simulink model "variableFrequencyConverter"  (R2021b)
settings: Solver=ode23tb  StartTime=simCtrl.startTime  StopTime=simCtrl.endTime  FixedStep=5e-7  RelTol=1e-3  EnableMultiTasking=on
values from neighbouring files (symbols this model uses):
  PhaseA_Grid_Amplitude = sqrt(2)*Vnet / sqrt(3)    [init.m]
  PhaseA_Grid_Bias = 0    [init.m]
  PhaseA_Grid_Frequency = 2*pi*fnet    [init.m]
  PhaseA_Grid_Phase = 0    [init.m]
  PhaseB_Grid_Amplitude = sqrt(2)*Vnet / sqrt(3)    [init.m]
  PhaseB_Grid_Bias = 0    [init.m]
  PhaseB_Grid_Frequency = 2*pi*fnet    [init.m]
  PhaseB_Grid_Phase = -2*pi/3    (= -2.09439510239)    [init.m]
  PhaseC_Grid_Amplitude = sqrt(2)*Vnet / sqrt(3)    [init.m]
  PhaseC_Grid_Bias = 0    [init.m]
  PhaseC_Grid_Frequency = 2*pi*fnet    [init.m]
  PhaseC_Grid_Phase = -4*pi/3    (= -4.18879020479)    [init.m]
  R_Convergence = (motor.un*1000)/(motor.In*sqrt(2))    [init.m]
  TcuP = -1 * TcuP    (= 0)    [init.m]
  TlinP = -1 * TlinP    (= 0)    [init.m]
  TsqP = -1 * TsqP    (= -1)    [init.m]
undefined symbols (not defined in the file or in its folder): ctrl, motor
libraries: spsDiodeLib x6, spsIGBTDiodeLib x6, powerlib_extras x4, spsSeriesRLCBranchLib x4, spsVoltageMeasurementLib x4, spsControlledVoltageSourceLib x3, spsControlledCurrentSourceLib x3, simulink x3, spsThreePhaseVIMeasurementLib x3, spsGroundLib x1, spsTriangleGeneratorLib x1, spspowerguiLib x1
settings Model: ModifiedByFormat=Aravindh Vishnu  Creator=Aravindh Vishnu  LastModifiedBy=Aravindh Vishnu
settings SolverCC: AlgebraicLoopSolver=TrustRegion
settings DataIOCC: FinalStateName=state_p3  InitialState=state_p3  SaveFormat=Array  SignalLoggingSaveFormat=ModelDataLogs  SaveOutput=off  SignalLogging=off  SaveTime=off  ReturnWorkspaceOutputs=off  SignalLoggingName=sigsOut
settings OptimizationCC: BlockReduction=off  DefaultParameterBehavior=Inlined  InlineInvariantSignals=on  BufferReuse=off  ExpressionDepthLimit=2147483647  InitFltsAndDblsToZero=on  LifeSpan=inf
settings DebuggingCC: SaveWithParameterizedLinksMsg=none  UnderspecifiedInitializationDetection=Classic  MergeDetectMultiDrivingBlocksExec=none  SignalResolutionControl=TryResolveAllWithWarning  MultiTaskDSMMsg=warning  MultiTaskCondExecSysMsg=none  FcnCallInpInsideContextMsg=warning  StateNameClashWarn=warning  SFUnexpectedBacktrackingDiag=warning  SFNoUnconditionalDefaultTransitionDiag=warning  SFExecutionAtInitializationDiag=none  SFMachineParentedDataDiag=warning  ArithmeticOperatorsInVariantConditions=warning
settings HardwareCC: ProdBitPerPointer=32  ProdBitPerSizeT=32  ProdBitPerPtrDiffT=32  ProdLargestAtomicFloat=None  ProdIntDivRoundTo=Undefined  ProdEndianess=Unspecified  ProdWordSize=32  ProdHWDeviceType=Generic->32-bit Real-Time Simulator  TargetBitPerPointer=64  TargetBitPerSizeT=64  TargetBitPerPtrDiffT=64  TargetLongLongMode=on  TargetIntDivRoundTo=Zero  TargetEndianess=LittleEndian  TargetWordSize=64  TargetHWDeviceType=MATLAB Host  ProdEqTarget=off
settings ModelReferenceCC: PropagateSignalLabelsOutOfModel=off
settings SFSimCC: SimUseLocalCustomCode=off  SimParseCustomCode=off  CustomCodeUndefinedFunction=UseInterfaceOnly
settings RTWCC: RTWUseLocalCustomCode=off
settings CodeAppCC: StateflowObjectComments=on
settings GRTTargetCC: TargetFcnLib=ansi_tfl_tmw.mat  TargetLangStandard=C89/C90 (ANSI)  CombineOutputUpdateFcns=off  GRTInterface=on
settings ConfigComp: CovMetricSettings=dw  CovSaveCumulativeToWorkspaceVar=on  CovSaveSingleToWorkspaceVar=on  CovExternalEMLEnable=off  CovSFcnEnable=off
settings SimscapeCC: SimscapeNormalizeSystem=off

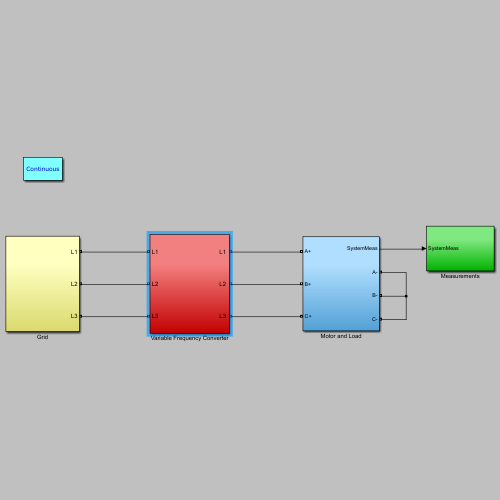
[thumbnail: Simulink's stored preview of the top-level diagram]
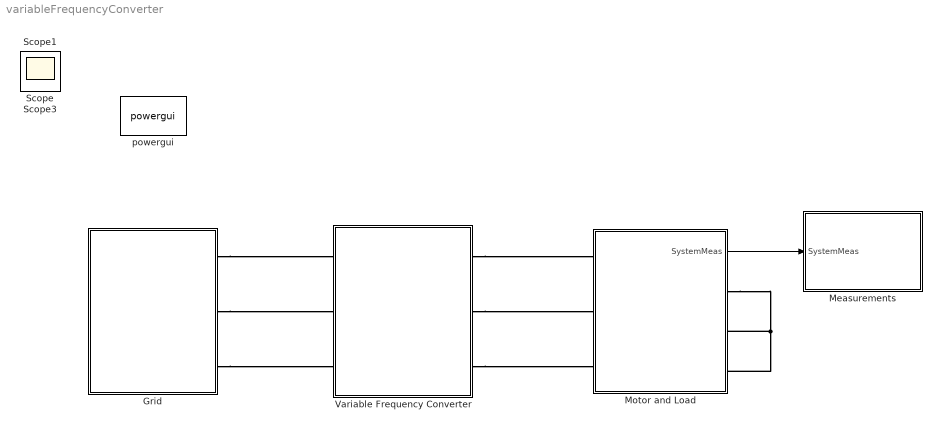
== system variableFrequencyConverter ==
  Grid : Subsystem
  Measurements : Subsystem
  Motor and Load : Subsystem
  Variable Frequency Converter : Subsystem
  powergui : spspowerguiLib/powergui  Priority=1  SimulationMode=Continuous  SampleTime=50e-6  frequency=60  Iterations=50  frequencyindice=0  Pbase=100e6  ErrMax=1e-4  UnitsV=kV  UnitsW=MW  buscounter=0  FunctionMessages=off  echomessages=off  EnableUseOfTLC=off  CurrentSourceSwitches=on  DisableSnubberDevices=off  DisableRonSwitches=off  DisableVfSwitches=off  DisplayEquations=off  AutomaticDiscreteSolvers=off  SolverType=Tustin  Interpol=off  ExternalGateDelay=off  methode=off  Ts=0  x0status=blocks  SPID=off  SwTol=0  HookPort=off  NonlinearTolerance=1e-4  nMaxIteration=100  ContinueOnMaxIteration=off  RestoreLinks=warning  ResistiveCurrentMeasurement=off  Frange=[0:2:500]  Ylog=off  Xlog=on  ShowGrid=off  save=off  variable=ZData  structure=0  ZoomFFT=on  StartTime=0.0  cycles=1  DisplayStyle=1  fundamental=60  FreqAxis=off  MaxFrequency=1000  frequencyindicesteady=1  RmsSteady=1  display=off
  Scope : Scope
  Scope1 : Scope
  Scope3 : Scope
  wires:
  Motor and Load/1(SystemMeas) -> Measurements/1(SystemMeas)
  connections:
  Motor and Load/RConn2 -- Motor and Load/RConn1 -- Motor and Load/RConn3
  Grid/RConn1 -- Variable Frequency Converter/LConn1
  Grid/RConn2 -- Variable Frequency Converter/LConn2
  Grid/RConn3 -- Variable Frequency Converter/LConn3
  Variable Frequency Converter/RConn3 -- Motor and Load/LConn3
  Variable Frequency Converter/RConn2 -- Motor and Load/LConn2
  Variable Frequency Converter/RConn1 -- Motor and Load/LConn1

== system variableFrequencyConverter/Grid ==
  Three phase power supply : Subsystem
  L1 : PMIOPort  Side=Right
  L2 : PMIOPort  Port=2  Side=Right
  L3 : PMIOPort  Port=3  Side=Right
  connections:
  Three phase power supply/RConn1 -- L1/RConn1
  Three phase power supply/RConn2 -- L2/RConn1
  Three phase power supply/RConn3 -- L3/RConn1

== system variableFrequencyConverter/Measurements ==
  SystemMeas : Inport
  Bus Selector1 : BusSelector  OutputSignals=V_s_abc,I_s_abc,Te,wm,rpm,T_load,slip,r_angle
  Mux : Mux  Inputs=2
  Oscilloscope 1 : Scope  NumInputPorts=2
  Oscilloscope 2 : Scope  NumInputPorts=2
  Oscilloscope 3 : Scope  NumInputPorts=3
  SystemMeas computations : Subsystem
  Terminator : Terminator
  Terminator1 : Terminator
  Terminator2 : Terminator
  wires:
  SystemMeas/1 -> Bus Selector1/1
  Bus Selector1/1 -> Oscilloscope 1/1  "<V_s_abc>"
  Bus Selector1/2 -> Oscilloscope 1/2  "<I_s_abc>"
  Bus Selector1/3 -> SystemMeas computations/1(Te), Oscilloscope 3/2  "<Te>"
  Bus Selector1/5 -> SystemMeas computations/2(Rpm), Oscilloscope 3/1  "<rpm>"
  Bus Selector1/6 -> Mux/2  "<T_load>"
  Bus Selector1/7 -> Terminator/1  "<slip>"
  Bus Selector1/8 -> Terminator1/1  "<r_angle>"
  Mux/1 -> Oscilloscope 3/3
  SystemMeas computations/1(Te_mean [Nm]) -> Mux/1
  SystemMeas computations/2(Te_mean [pu]) -> Oscilloscope 2/1
  SystemMeas computations/3(rpm [pu]) -> Oscilloscope 2/2
  Bus Selector1/4 -> Terminator2/1  "<wm>"

== system variableFrequencyConverter/Motor and Load ==
  Bus Creator : BusCreator  Inputs=8
  Induction motor open stator winding : Subsystem
  Load model : Subsystem
  Measurements selector : Subsystem
  A+ : PMIOPort  Side=Left
  B+ : PMIOPort  Port=2  Side=Left
  C+ : PMIOPort  Port=3  Side=Left
  A- : PMIOPort  Port=4  Side=Right
  B- : PMIOPort  Port=5  Side=Right
  C- : PMIOPort  Port=6  Side=Right
  SystemMeas : Outport  VectorParamsAs1DForOutWhenUnconnected=off
  wires:
  Induction motor open stator winding/1(m) -> Measurements selector/1(m)
  Bus Creator/1 -> SystemMeas/1
  Load model/1(Tm) -> Induction motor open stator winding/1(Tm)
  Measurements selector/1(wm) -> Bus Creator/1, Load model/1(wm)  "wm"
  Measurements selector/2(V_s_abc) -> Bus Creator/2  "V_s_abc"
  Measurements selector/3(I_s_abc) -> Bus Creator/3  "I_s_abc"
  Measurements selector/4(Te) -> Bus Creator/4  "Te"
  Measurements selector/5(slip) -> Bus Creator/5  "slip"
  Measurements selector/6(r_angle) -> Bus Creator/6  "r_angle"
  Measurements selector/7(T_load) -> Bus Creator/7  "T_load"
  Measurements selector/8(rpm) -> Bus Creator/8  "rpm"
  connections:
  Induction motor open stator winding/RConn2 -- B-/RConn1
  Induction motor open stator winding/RConn3 -- C-/RConn1
  B+/RConn1 -- Induction motor open stator winding/LConn2
  Induction motor open stator winding/RConn1 -- A-/RConn1
  A+/RConn1 -- Induction motor open stator winding/LConn1
  C+/RConn1 -- Induction motor open stator winding/LConn3

== system variableFrequencyConverter/Variable Frequency Converter ==
  " Scope5" : Scope  NumInputPorts=3
  Controller : Subsystem
  Load Measurement : Subsystem
  Power Electronics Module : Subsystem
  L1 : PMIOPort  Side=Left
  L2 : PMIOPort  Port=2  Side=Left
  "L1 " : PMIOPort  Port=3  Side=Right
  "L2 " : PMIOPort  Port=4  Side=Right
  L3 : PMIOPort  Port=5  Side=Left
  "L3 " : PMIOPort  Port=6  Side=Right
  wires:
  Controller/1(gateSignals) -> Power Electronics Module/1(gateSignals)
  Load Measurement/1(iload) -> " Scope5"/1, Controller/1(current)
  Load Measurement/2(UL_load) -> " Scope5"/2
  Load Measurement/3(uL_load) -> " Scope5"/3
  connections:
  L1/RConn1 -- Power Electronics Module/LConn1
  L2/RConn1 -- Power Electronics Module/LConn2
  L3/RConn1 -- Power Electronics Module/LConn3
  Power Electronics Module/RConn1 -- Load Measurement/LConn1
  Power Electronics Module/RConn2 -- Load Measurement/LConn2
  Power Electronics Module/RConn3 -- Load Measurement/LConn3
  Load Measurement/RConn3 -- "L3 "/RConn1
  Load Measurement/RConn2 -- "L2 "/RConn1
  Load Measurement/RConn1 -- "L1 "/RConn1

== system variableFrequencyConverter/Grid/Three phase power supply ==
  Controlled Voltage Source phase L1 : spsControlledVoltageSourceLib/Controlled Voltage Source  Initialize=off  Source_Type=AC  Amplitude=0  Phase=0  Frequency=0  Measurements=None
  Controlled Voltage Source phase L2 : spsControlledVoltageSourceLib/Controlled Voltage Source  Initialize=off  Source_Type=AC  Amplitude=0  Phase=0  Frequency=0  Measurements=None
  Controlled Voltage Source phase L3 : spsControlledVoltageSourceLib/Controlled Voltage Source  Initialize=off  Source_Type=AC  Amplitude=0  Phase=0  Frequency=0  Measurements=None
  Ground3 : spsGroundLib/Ground  LConnTagsString=a
  Sine Wave Phase A : Sin  Amplitude=PhaseA_Grid_Amplitude  Bias=PhaseA_Grid_Bias  Frequency=PhaseA_Grid_Frequency  Phase=PhaseA_Grid_Phase  SampleTime=0
  Sine Wave Phase B : Sin  Amplitude=PhaseB_Grid_Amplitude  Bias=PhaseB_Grid_Bias  Frequency=PhaseB_Grid_Frequency  Phase=PhaseB_Grid_Phase  SampleTime=0
  Sine Wave Phase C : Sin  Amplitude=PhaseC_Grid_Amplitude  Bias=PhaseC_Grid_Bias  Frequency=PhaseC_Grid_Frequency  Phase=PhaseC_Grid_Phase  SampleTime=0
  L1 : PMIOPort  Side=Right
  L2 : PMIOPort  Port=2  Side=Right
  L3 : PMIOPort  Port=3  Side=Right
  wires:
  Sine Wave Phase A/1 -> Controlled Voltage Source phase L1/1
  Sine Wave Phase B/1 -> Controlled Voltage Source phase L2/1
  Sine Wave Phase C/1 -> Controlled Voltage Source phase L3/1
  connections:
  Controlled Voltage Source phase L3/LConn1 -- Ground3/LConn1 -- Controlled Voltage Source phase L1/LConn1 -- Controlled Voltage Source phase L2/LConn1
  L2/RConn1 -- Controlled Voltage Source phase L2/RConn1
  L3/RConn1 -- Controlled Voltage Source phase L3/RConn1
  L1/RConn1 -- Controlled Voltage Source phase L1/RConn1

== system variableFrequencyConverter/Measurements/SystemMeas computations ==
  Te : Inport
  Rpm : Inport  Port=2
  Mean Value : powerlib_extras/Measurements/Mean Value  Period=1/motor.fn
      settings: SourceProductBaseCode=PS
  Te_mean/T_base : Gain  Gain=1/motor.Tl_nom
  rpm/rpm_synch : Gain  Gain=1/((60*motor.wb)/(2*pi*motor.np))
  Te_mean [Nm] : Outport  VectorParamsAs1DForOutWhenUnconnected=off
  Te_mean [pu] : Outport  Port=2  VectorParamsAs1DForOutWhenUnconnected=off
  rpm [pu] : Outport  Port=3  VectorParamsAs1DForOutWhenUnconnected=off
  wires:
  Te/1 -> Mean Value/1
  Mean Value/1 -> Te_mean/T_base/1, Te_mean [Nm]/1
  Te_mean/T_base/1 -> Te_mean [pu]/1
  Rpm/1 -> rpm/rpm_synch/1
  rpm/rpm_synch/1 -> rpm [pu]/1

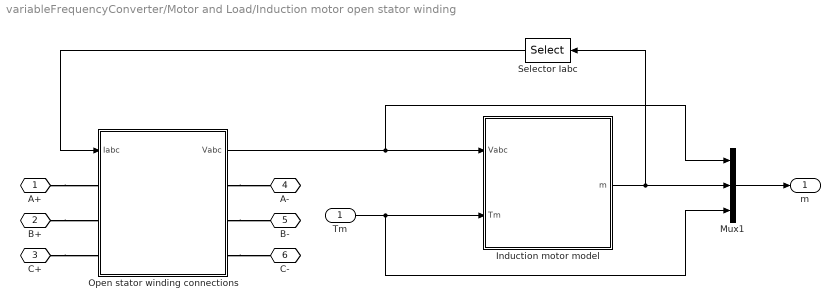
== system variableFrequencyConverter/Motor and Load/Induction motor open stator winding ==
  Tm : Inport
  Induction motor model : Subsystem
  Mux1 : Mux  Inputs=3
  Open stator winding connections : Subsystem
  Selector Iabc : Selector  InputPortWidth=8  IndexOptions=Index vector (dialog)  Indices=[1 2 3]  OutputSizes=1
  A+ : PMIOPort  Side=Left
  B+ : PMIOPort  Port=2  Side=Left
  C+ : PMIOPort  Port=3  Side=Left
  A- : PMIOPort  Port=4  Side=Right
  B- : PMIOPort  Port=5  Side=Right
  C- : PMIOPort  Port=6  Side=Right
  m : Outport  VectorParamsAs1DForOutWhenUnconnected=off
  wires:
  Open stator winding connections/1(Vabc) -> Mux1/1, Induction motor model/1(Vabc)
  Tm/1 -> Mux1/3, Induction motor model/2(Tm)
  Induction motor model/1(m) -> Selector Iabc/1, Mux1/2
  Selector Iabc/1 -> Open stator winding connections/1(Iabc)
  Mux1/1 -> m/1
  connections:
  A+/RConn1 -- Open stator winding connections/LConn1
  B+/RConn1 -- Open stator winding connections/LConn2
  C+/RConn1 -- Open stator winding connections/LConn3
  Open stator winding connections/RConn1 -- A-/RConn1
  Open stator winding connections/RConn2 -- B-/RConn1
  Open stator winding connections/RConn3 -- C-/RConn1

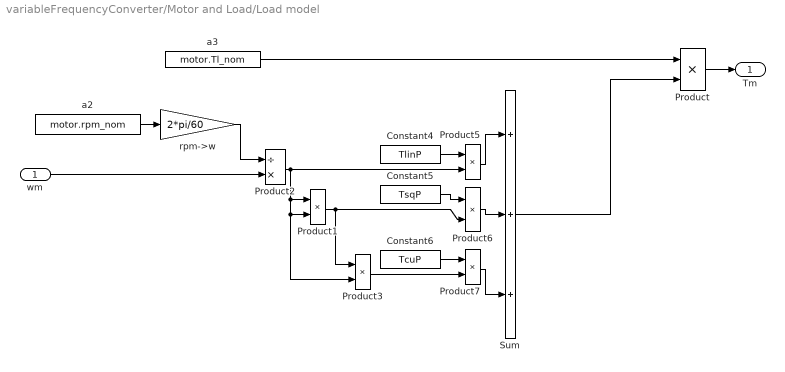
== system variableFrequencyConverter/Motor and Load/Load model ==
  wm : Inport
  Constant4 : Constant  Value=TlinP
  Constant5 : Constant  Value=TsqP
  Constant6 : Constant  Value=TcuP
  Product{,1,3,5..7} (6 alike) : Product  SaturateOnIntegerOverflow=on  OutDataTypeStr=Inherit: Same as first input
  Product2 : Product  Inputs=/*  SaturateOnIntegerOverflow=on  OutDataTypeStr=Inherit: Same as first input
  Sum : Sum  Inputs=+++  SaturateOnIntegerOverflow=on
  a2 : Constant  Value=motor.rpm_nom
  a3 : Constant  Value=motor.Tl_nom
  rpm->w : Gain  Gain=2*pi/60  SaturateOnIntegerOverflow=on  OutDataTypeStr=Inherit: Same as input  ParamDataTypeStr=Inherit: Same as input
  Tm : Outport  VectorParamsAs1DForOutWhenUnconnected=off
  wires:
  Product/1 -> Tm/1
  wm/1 -> Product2/2
  rpm->w/1 -> Product2/1
  Product2/1 -> Product1/1, Product1/2, Product3/2, Product5/2
  Product1/1 -> Product3/1, Product6/2
  Constant4/1 -> Product5/1
  Constant5/1 -> Product6/1
  Constant6/1 -> Product7/1
  Product3/1 -> Product7/2
  a3/1 -> Product/1
  a2/1 -> rpm->w/1
  Product5/1 -> Sum/1
  Product6/1 -> Sum/2
  Product7/1 -> Sum/3
  Sum/1 -> Product/2

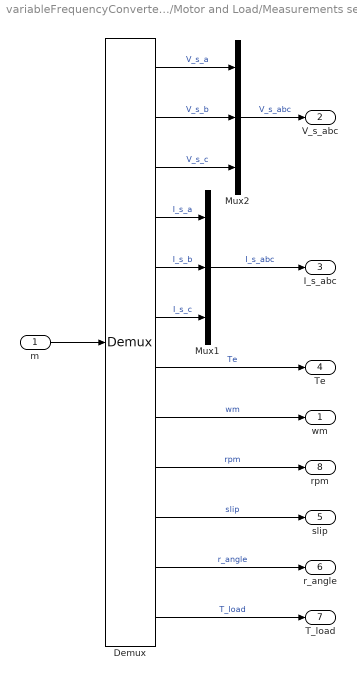
== system variableFrequencyConverter/Motor and Load/Measurements selector ==
  m : Inport
  Demux : Demux  Outputs=12
      settings: DisplayOption=none
  Mux1 : Mux  Inputs=3
  Mux2 : Mux  Inputs=3
  wm : Outport  VectorParamsAs1DForOutWhenUnconnected=off
  V_s_abc : Outport  Port=2  VectorParamsAs1DForOutWhenUnconnected=off
  I_s_abc : Outport  Port=3  VectorParamsAs1DForOutWhenUnconnected=off
  Te : Outport  Port=4  VectorParamsAs1DForOutWhenUnconnected=off
  slip : Outport  Port=5  VectorParamsAs1DForOutWhenUnconnected=off
  r_angle : Outport  Port=6  VectorParamsAs1DForOutWhenUnconnected=off
  T_load : Outport  Port=7  VectorParamsAs1DForOutWhenUnconnected=off
  rpm : Outport  Port=8  VectorParamsAs1DForOutWhenUnconnected=off
  wires:
  Mux1/1 -> I_s_abc/1  "I_s_abc"
  Mux2/1 -> V_s_abc/1  "V_s_abc"
  m/1 -> Demux/1
  Demux/1 -> Mux2/1  "V_s_a"
  Demux/3 -> Mux2/3  "V_s_c"
  Demux/2 -> Mux2/2  "V_s_b"
  Demux/4 -> Mux1/1  "I_s_a"
  Demux/5 -> Mux1/2  "I_s_b"
  Demux/6 -> Mux1/3  "I_s_c"
  Demux/7 -> Te/1  "Te"
  Demux/8 -> wm/1  "wm"
  Demux/9 -> rpm/1  "rpm"
  Demux/10 -> slip/1  "slip"
  Demux/11 -> r_angle/1  "r_angle"
  Demux/12 -> T_load/1  "T_load"

== system variableFrequencyConverter/Variable Frequency Converter/Controller ==
  current : Inport
  Clock : Clock
  ControlProcess : Subsystem
  PwmDriver : Subsystem
  deltaControlProcess : DiscretePulseGenerator  PulseType=Time based  Period=ctrl.deltaControlProcess  PulseWidth=50
  gateSignals : Outport  VectorParamsAs1DForOutWhenUnconnected=off
  wires:
  current/1 -> ControlProcess/1(current)
  Clock/1 -> ControlProcess/2(time)
  ControlProcess/1(ccrValues) -> PwmDriver/1(ccrValues)
  PwmDriver/1(gateSignals) -> gateSignals/1
  deltaControlProcess/1 -> ControlProcess/Trigger

== system variableFrequencyConverter/Variable Frequency Converter/Load Measurement ==
  Load P2N V measurement : spsThreePhaseVIMeasurementLib/Three-Phase V-I Measurement  VoltageMeasurement=phase-to-ground  SetLabelV=off  LabelV=L123  Vpu=off  VpuLL=off  CurrentMeasurement=no  SetLabelI=off  LabelI=Iabc  Ipu=off  Pbase=100e6  Vbase=500e3  OutputType=Complex  PhasorSimulation=off  PSBequivalent=0
  Load P2P V measurement : spsThreePhaseVIMeasurementLib/Three-Phase V-I Measurement  VoltageMeasurement=phase-to-phase  SetLabelV=off  LabelV=L123  Vpu=off  VpuLL=off  CurrentMeasurement=yes  SetLabelI=off  LabelI=Iabc  Ipu=off  Pbase=100e6  Vbase=500e3  OutputType=Complex  PhasorSimulation=off  PSBequivalent=0
  L1 : PMIOPort  Side=Left
  L2 : PMIOPort  Port=2  Side=Left
  L3 : PMIOPort  Port=3  Side=Left
  "L1 " : PMIOPort  Port=4  Side=Right
  "L2 " : PMIOPort  Port=5  Side=Right
  "L3 " : PMIOPort  Port=6  Side=Right
  iload : Outport  VectorParamsAs1DForOutWhenUnconnected=off
  UL_load : Outport  Port=2  VectorParamsAs1DForOutWhenUnconnected=off
  uL_load : Outport  Port=3  VectorParamsAs1DForOutWhenUnconnected=off
  wires:
  Load P2N V measurement/1 -> uL_load/1
  Load P2P V measurement/1 -> UL_load/1
  Load P2P V measurement/2 -> iload/1
  connections:
  L1/RConn1 -- Load P2N V measurement/LConn1
  L2/RConn1 -- Load P2N V measurement/LConn2
  L3/RConn1 -- Load P2N V measurement/LConn3
  Load P2N V measurement/RConn1 -- Load P2P V measurement/LConn1
  Load P2N V measurement/RConn2 -- Load P2P V measurement/LConn2
  Load P2N V measurement/RConn3 -- Load P2P V measurement/LConn3
  Load P2P V measurement/RConn1 -- "L1 "/RConn1
  Load P2P V measurement/RConn2 -- "L2 "/RConn1
  Load P2P V measurement/RConn3 -- "L3 "/RConn1

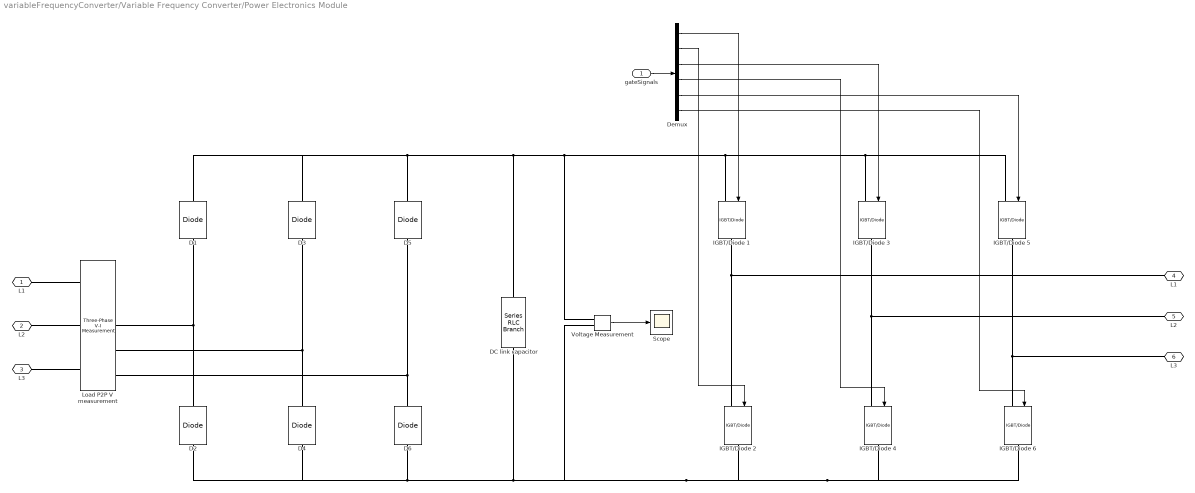
== system variableFrequencyConverter/Variable Frequency Converter/Power Electronics Module ==
  gateSignals : Inport
  " Scope" : Scope
  D{1..6} (6 alike) : spsDiodeLib/Diode  Ron=0.001  Lon=0  Vf=0.8  IC=0  UseSnubber=off  Rs=500  Cs=250e-9  Measurements=off
  DC link capacitor : spsSeriesRLCBranchLib/Series RLC Branch  LConnTagsString=__new0  RConnTagsString=__new0  BranchType=C  Resistance=1  Inductance=1e-3  SetiL0=off  InitialCurrent=0  Capacitance=10000e-6  Setx0=off  InitialVoltage=507  Measurements=None
  Demux : Demux  Outputs=6
  IGBT/Diode {1..6} (6 alike) : spsIGBTDiodeLib/IGBT//Diode  Ron=1e-3  Rs=1e5  Cs=inf  Measurements=off
  Load P2P V measurement : spsThreePhaseVIMeasurementLib/Three-Phase V-I Measurement  VoltageMeasurement=phase-to-ground  SetLabelV=off  LabelV=L123  Vpu=off  VpuLL=off  CurrentMeasurement=yes  SetLabelI=off  LabelI=Iabc  Ipu=off  Pbase=100e6  Vbase=500e3  OutputType=Complex  PhasorSimulation=off  PSBequivalent=0
  Voltage Measurement : spsVoltageMeasurementLib/Voltage Measurement  PhasorSimulation=off  OutputType=Complex  PSBequivalent=0
  L1 : PMIOPort  Side=Left
  L2 : PMIOPort  Port=2  Side=Left
  L3 : PMIOPort  Port=3  Side=Left
  "L1 " : PMIOPort  Port=4  Side=Right
  "L2 " : PMIOPort  Port=5  Side=Right
  "L3 " : PMIOPort  Port=6  Side=Right
  wires:
  gateSignals/1 -> Demux/1
  Voltage Measurement/1 -> " Scope"/1
  Demux/1 -> IGBT/Diode 1/1
  Demux/2 -> IGBT/Diode 2/1
  Demux/3 -> IGBT/Diode 3/1
  Demux/4 -> IGBT/Diode 4/1
  Demux/5 -> IGBT/Diode 5/1
  Demux/6 -> IGBT/Diode 6/1
  connections:
  D2/RConn1 -- Load P2P V measurement/RConn1 -- D1/LConn1
  D4/RConn1 -- Load P2P V measurement/RConn2 -- D3/LConn1
  D6/RConn1 -- Load P2P V measurement/RConn3 -- D5/LConn1
  IGBT/Diode 1/RConn1 -- IGBT/Diode 2/LConn1 -- "L1 "/RConn1
  IGBT/Diode 4/LConn1 -- "L2 "/RConn1 -- IGBT/Diode 3/RConn1
  IGBT/Diode 6/LConn1 -- "L3 "/RConn1 -- IGBT/Diode 5/RConn1
  L1/RConn1 -- Load P2P V measurement/LConn1
  L2/RConn1 -- Load P2P V measurement/LConn2
  L3/RConn1 -- Load P2P V measurement/LConn3
  D4/LConn1 -- D2/LConn1 -- DC link capacitor/RConn1 -- IGBT/Diode 2/RConn1 -- IGBT/Diode 6/RConn1 -- IGBT/Diode 4/RConn1 -- Voltage Measurement/LConn2 -- D6/LConn1
  D1/RConn1 -- D3/RConn1 -- DC link capacitor/LConn1 -- Voltage Measurement/LConn1 -- IGBT/Diode 1/LConn1 -- IGBT/Diode 3/LConn1 -- IGBT/Diode 5/LConn1 -- D5/RConn1

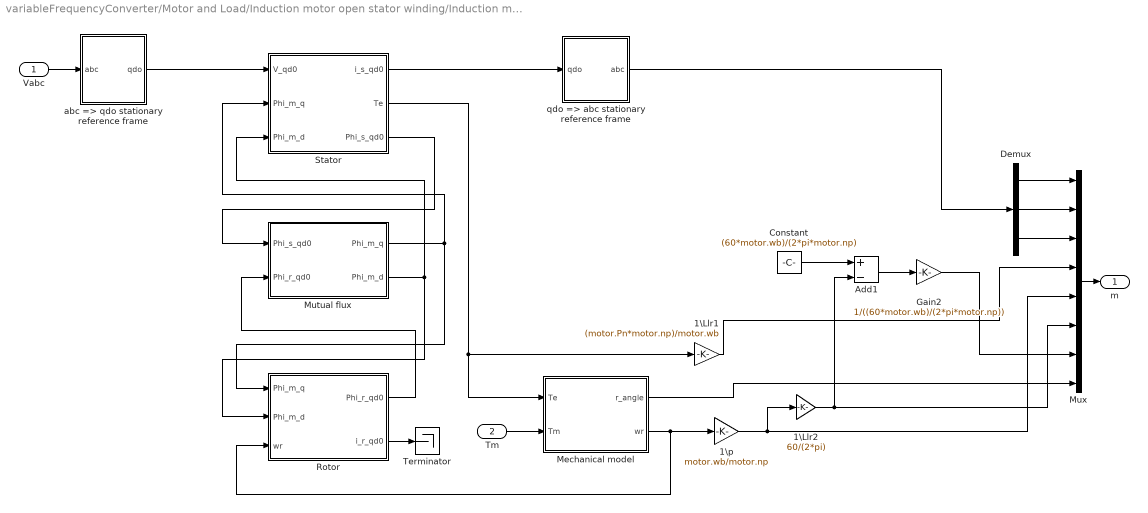
== system variableFrequencyConverter/Motor and Load/Induction motor open stator winding/Induction motor model ==
  Vabc : Inport
  Tm : Inport  Port=2
  1\Llr1 : Gain  Gain=(motor.Pn*motor.np)/motor.wb  SaturateOnIntegerOverflow=on  OutDataTypeStr=Inherit: Same as input  ParamDataTypeStr=Inherit: Same as input
  1\Llr2 : Gain  Gain=60/(2*pi)  SaturateOnIntegerOverflow=on  OutDataTypeStr=Inherit: Same as input  ParamDataTypeStr=Inherit: Same as input
  1\p : Gain  Gain=motor.wb/motor.np  SaturateOnIntegerOverflow=on  OutDataTypeStr=Inherit: Same as input  ParamDataTypeStr=Inherit: Same as input
  Add1 : Sum  Inputs=+-
  Constant : Constant  Value=(60*motor.wb)/(2*pi*motor.np)
  Demux : Demux  Outputs=3
  Gain2 : Gain  Gain=1/((60*motor.wb)/(2*pi*motor.np))
  Mechanical model : Subsystem
  Mutual flux : Subsystem
  Mux : Mux  Inputs=8
  Rotor : Subsystem
  Stator : Subsystem
  Terminator : Terminator
  abc => qdo stationary reference frame : Subsystem
  qdo => abc stationary reference frame : Subsystem
  m : Outport  VectorParamsAs1DForOutWhenUnconnected=off
  wires:
  Mutual flux/1(Phi_m_q) -> Stator/2(Phi_m_q), Rotor/1(Phi_m_q)
  Mutual flux/2(Phi_m_d) -> Rotor/2(Phi_m_d), Stator/3(Phi_m_d)
  Rotor/1(Phi_r_qd0) -> Mutual flux/2(Phi_r_qd0)
  Stator/3(Phi_s_qd0) -> Mutual flux/1(Phi_s_qd0)
  Vabc/1 -> abc => qdo stationary reference frame/1(abc)
  abc => qdo stationary reference frame/1(qdo) -> Stator/1(V_qd0)
  Stator/1(i_s_qd0) -> qdo => abc stationary reference frame/1(qdo)
  Stator/2(Te) -> Mechanical model/1(Te), 1\Llr1/1
  Mechanical model/2(wr) -> 1\p/1, Rotor/3(wr)
  Tm/1 -> Mechanical model/2(Tm)
  1\p/1 -> 1\Llr2/1, Mux/5
  1\Llr2/1 -> Mux/6, Add1/2
  Add1/1 -> Gain2/1
  Constant/1 -> Add1/1
  Mux/1 -> m/1
  qdo => abc stationary reference frame/1(abc) -> Demux/1
  Demux/1 -> Mux/1
  Demux/2 -> Mux/2
  Demux/3 -> Mux/3
  1\Llr1/1 -> Mux/4
  Gain2/1 -> Mux/7
  Mechanical model/1(r_angle) -> Mux/8
  Rotor/2(i_r_qd0) -> Terminator/1

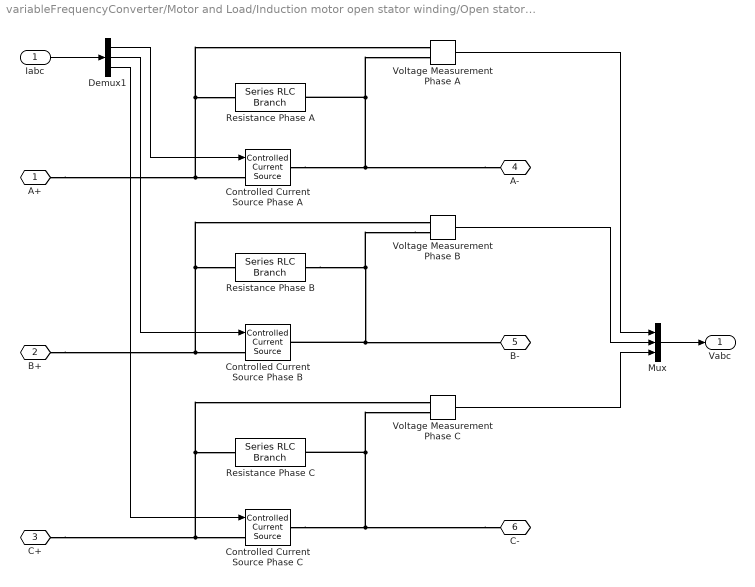
== system variableFrequencyConverter/Motor and Load/Induction motor open stator winding/Open stator winding connections ==
  Iabc : Inport
  Controlled Current Source Phase A : spsControlledCurrentSourceLib/Controlled Current Source  Initialize=off  Source_Type=AC  Amplitude=0  Phase=0  Frequency=0  Measurements=None
  Controlled Current Source Phase B : spsControlledCurrentSourceLib/Controlled Current Source  Initialize=off  Source_Type=AC  Amplitude=0  Phase=0  Frequency=0  Measurements=None
  Controlled Current Source Phase C : spsControlledCurrentSourceLib/Controlled Current Source  Initialize=off  Source_Type=AC  Amplitude=0  Phase=0  Frequency=0  Measurements=None
  Demux1 : Demux  Outputs=3
  Mux : Mux  Inputs=3
  Resistance Phase A : spsSeriesRLCBranchLib/Series RLC Branch  LConnTagsString=__new0  RConnTagsString=__new0  BranchType=R  Resistance=R_Convergence  Inductance=1e-3  SetiL0=off  InitialCurrent=0  Capacitance=1e-6  Setx0=off  InitialVoltage=0  Measurements=None
  Resistance Phase B : spsSeriesRLCBranchLib/Series RLC Branch  LConnTagsString=__new0  RConnTagsString=__new0  BranchType=R  Resistance=R_Convergence  Inductance=1e-3  SetiL0=off  InitialCurrent=0  Capacitance=1e-6  Setx0=off  InitialVoltage=0  Measurements=None
  Resistance Phase C : spsSeriesRLCBranchLib/Series RLC Branch  LConnTagsString=__new0  RConnTagsString=__new0  BranchType=R  Resistance=R_Convergence  Inductance=1e-3  SetiL0=off  InitialCurrent=0  Capacitance=1e-6  Setx0=off  InitialVoltage=0  Measurements=None
  Voltage Measurement Phase A : spsVoltageMeasurementLib/Voltage Measurement  PhasorSimulation=off  OutputType=Complex  PSBequivalent=0
  Voltage Measurement Phase B : spsVoltageMeasurementLib/Voltage Measurement  PhasorSimulation=off  OutputType=Complex  PSBequivalent=0
  Voltage Measurement Phase C : spsVoltageMeasurementLib/Voltage Measurement  PhasorSimulation=off  OutputType=Complex  PSBequivalent=0
  A+ : PMIOPort  Side=Left
  B+ : PMIOPort  Port=2  Side=Left
  C+ : PMIOPort  Port=3  Side=Left
  A- : PMIOPort  Port=4  Side=Right
  B- : PMIOPort  Port=5  Side=Right
  C- : PMIOPort  Port=6  Side=Right
  Vabc : Outport  VectorParamsAs1DForOutWhenUnconnected=off
  wires:
  Iabc/1 -> Demux1/1
  Demux1/1 -> Controlled Current Source Phase A/1
  Demux1/2 -> Controlled Current Source Phase B/1
  Demux1/3 -> Controlled Current Source Phase C/1
  Mux/1 -> Vabc/1
  Voltage Measurement Phase A/1 -> Mux/1
  Voltage Measurement Phase B/1 -> Mux/2
  Voltage Measurement Phase C/1 -> Mux/3
  connections:
  A+/RConn1 -- Controlled Current Source Phase A/LConn1 -- Resistance Phase A/LConn1 -- Voltage Measurement Phase A/LConn1
  B+/RConn1 -- Controlled Current Source Phase B/LConn1 -- Resistance Phase B/LConn1 -- Voltage Measurement Phase B/LConn1
  C+/RConn1 -- Controlled Current Source Phase C/LConn1 -- Resistance Phase C/LConn1 -- Voltage Measurement Phase C/LConn1
  Voltage Measurement Phase B/LConn2 -- Resistance Phase B/RConn1 -- B-/RConn1 -- Controlled Current Source Phase B/RConn1
  A-/RConn1 -- Controlled Current Source Phase A/RConn1 -- Resistance Phase A/RConn1 -- Voltage Measurement Phase A/LConn2
  C-/RConn1 -- Controlled Current Source Phase C/RConn1 -- Resistance Phase C/RConn1 -- Voltage Measurement Phase C/LConn2

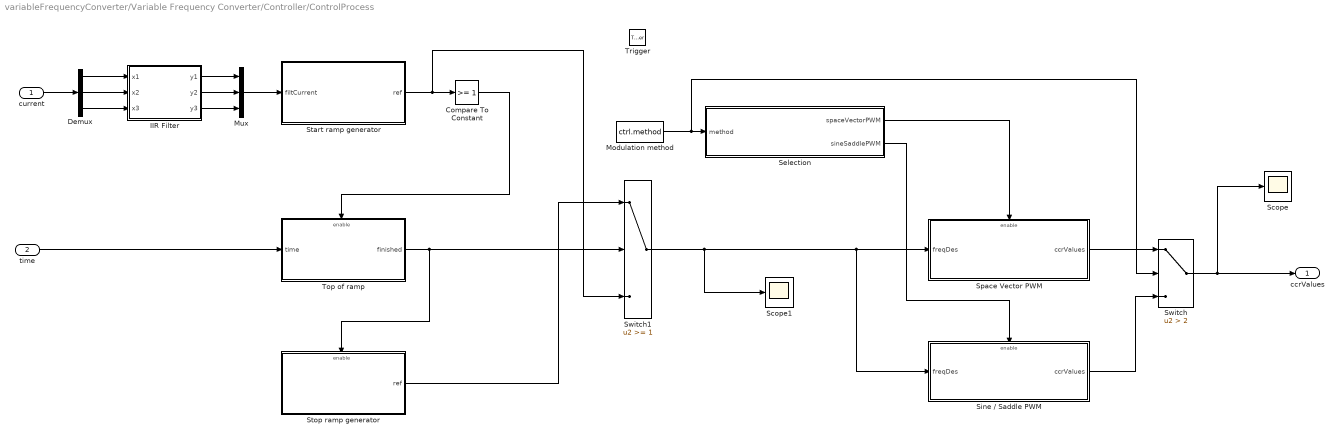
== system variableFrequencyConverter/Variable Frequency Converter/Controller/ControlProcess ==
  current : Inport
  time : Inport  Port=2
  Trigger : TriggerPort  VariantControl=(inherit)  PortDimensions=1
  " Scope" : Scope
  " Scope1" : Scope
  Compare To Constant : simulink/Logic and Bit Operations/Compare To Constant  relop=>=  const=1  OutDataTypeStr=boolean
  Demux : Demux  Outputs=3
  IIR Filter : MATLAB Function  TreatAsAtomicUnit=on
  Modulation method : Constant  Value=ctrl.method
  Mux : Mux  Inputs=3
  Selection : MATLAB Function  TreatAsAtomicUnit=on
  Sine / Saddle PWM : Subsystem
  Space Vector PWM : Subsystem  TreatAsAtomicUnit=on
  Start ramp generator : Subsystem
  Stop ramp generator : Subsystem
  Switch : Switch  Criteria=u2 > Threshold  Threshold=2
  Switch1 : Switch  Threshold=1
  Top of ramp : Subsystem
  ccrValues : Outport
  wires:
  Switch/1 -> ccrValues/1, " Scope"/1
  Selection/1(spaceVectorPWM) -> Space Vector PWM/Enable
  Switch1/1 -> " Scope1"/1, Sine / Saddle PWM/1(freqDes), Space Vector PWM/1(freqDes)
  current/1 -> Demux/1
  Demux/2 -> IIR Filter/2(x2)
  Demux/3 -> IIR Filter/3(x3)
  Top of ramp/1(finished) -> Switch1/2, Stop ramp generator/Enable
  Modulation method/1 -> Switch/2, Selection/1(method)
  Demux/1 -> IIR Filter/1(x1)
  IIR Filter/3(y3) -> Mux/3
  IIR Filter/1(y1) -> Mux/1
  IIR Filter/2(y2) -> Mux/2
  Start ramp generator/1(ref) -> Compare To Constant/1, Switch1/3
  Stop ramp generator/1(ref) -> Switch1/1
  Sine / Saddle PWM/1(ccrValues) -> Switch/3
  Selection/2(sineSaddlePWM) -> Sine / Saddle PWM/Enable
  Space Vector PWM/1(ccrValues) -> Switch/1
  Mux/1 -> Start ramp generator/1(filtCurrent)
  Compare To Constant/1 -> Top of ramp/Enable
  time/1 -> Top of ramp/1(time)

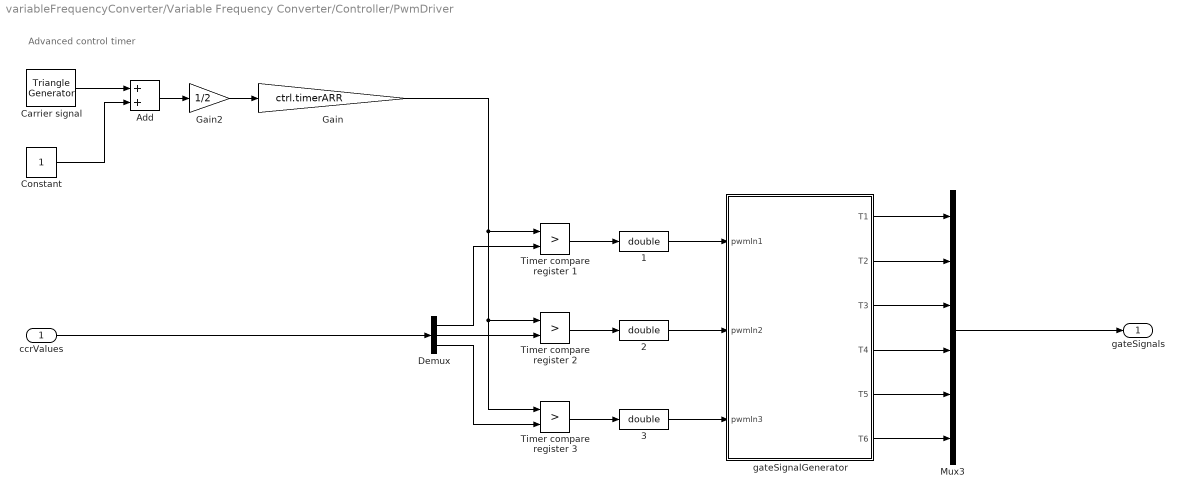
== system variableFrequencyConverter/Variable Frequency Converter/Controller/PwmDriver ==
  note: Advanced control timer
  ccrValues : Inport
  " 1" : DataTypeConversion  OutDataTypeStr=double
  " 2" : DataTypeConversion  OutDataTypeStr=double
  " 3" : DataTypeConversion  OutDataTypeStr=double
  Add : Sum
  Carrier signal : spsTriangleGeneratorLib/Triangle Generator  Freq=ctrl.pwmFrequency  Phase=0  Ts=0
  Constant : Constant
  Demux : Demux  Outputs=3
  Gain : Gain  Gain=ctrl.timerARR
  Gain2 : Gain  Gain=1/2
  Mux3 : Mux  Inputs=6
  Timer compare register 1 : RelationalOperator  Operator=>  OutDataTypeStr=boolean  RndMeth=Simplest
  Timer compare register 2 : RelationalOperator  Operator=>  OutDataTypeStr=boolean  RndMeth=Simplest
  Timer compare register 3 : RelationalOperator  Operator=>  OutDataTypeStr=boolean  RndMeth=Simplest
  gateSignalGenerator : MATLAB Function  TreatAsAtomicUnit=on
  gateSignals : Outport
  wires:
  Timer compare register 2/1 -> " 2"/1
  " 3"/1 -> gateSignalGenerator/3(pwmIn3)
  Demux/3 -> Timer compare register 3/2
  Timer compare register 3/1 -> " 3"/1
  Add/1 -> Gain2/1
  " 2"/1 -> gateSignalGenerator/2(pwmIn2)
  Demux/2 -> Timer compare register 2/2
  Constant/1 -> Add/2
  " 1"/1 -> gateSignalGenerator/1(pwmIn1)
  gateSignalGenerator/3(T3) -> Mux3/3
  Gain/1 -> Timer compare register 3/1, Timer compare register 2/1, Timer compare register 1/1
  Timer compare register 1/1 -> " 1"/1
  gateSignalGenerator/6(T6) -> Mux3/6
  gateSignalGenerator/1(T1) -> Mux3/1
  Carrier signal/1 -> Add/1
  Demux/1 -> Timer compare register 1/2
  gateSignalGenerator/2(T2) -> Mux3/2
  Gain2/1 -> Gain/1
  gateSignalGenerator/4(T4) -> Mux3/4
  gateSignalGenerator/5(T5) -> Mux3/5
  ccrValues/1 -> Demux/1
  Mux3/1 -> gateSignals/1

== system variableFrequencyConverter/Motor and Load/Induction motor open stator winding/Induction motor model/Mechanical model ==
  Te : Inport
  Tm : Inport  Port=2
  1\Llr2 : Gain  Gain=1/motor.Tb  SaturateOnIntegerOverflow=on  OutDataTypeStr=Inherit: Same as input  ParamDataTypeStr=Inherit: Same as input
  1\Llr3 : Gain  Gain=motor.wb  SaturateOnIntegerOverflow=on  OutDataTypeStr=Inherit: Same as input  ParamDataTypeStr=Inherit: Same as input
  1\p1 : Gain  Gain=1/motor.np  SaturateOnIntegerOverflow=on  OutDataTypeStr=Inherit: Same as input  ParamDataTypeStr=Inherit: Same as input
  1_2H1 : Gain  Gain=1/(2*motor.H)  SaturateOnIntegerOverflow=on  OutDataTypeStr=Inherit: Same as input  ParamDataTypeStr=Inherit: Same as input
  Add : Sum  Inputs=+--
  F1 : Gain  Gain=motor.b  SaturateOnIntegerOverflow=on  OutDataTypeStr=Inherit: Same as input  ParamDataTypeStr=Inherit: Same as input
  Rotor angle theta : Integrator
  Rotor angular velocity : Integrator
  r_angle : Outport  VectorParamsAs1DForOutWhenUnconnected=off
  wr : Outport  Port=2  VectorParamsAs1DForOutWhenUnconnected=off
  wires:
  Tm/1 -> 1\Llr2/1
  Te/1 -> Add/1
  Add/1 -> 1_2H1/1
  1_2H1/1 -> Rotor angular velocity/1
  Rotor angular velocity/1 -> 1\Llr3/1, F1/1, wr/1
  1\Llr3/1 -> Rotor angle theta/1
  1\Llr2/1 -> Add/2
  F1/1 -> Add/3
  Rotor angle theta/1 -> 1\p1/1
  1\p1/1 -> r_angle/1

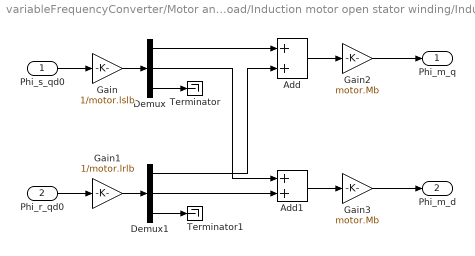
== system variableFrequencyConverter/Motor and Load/Induction motor open stator winding/Induction motor model/Mutual flux ==
  Phi_s_qd0 : Inport
  Phi_r_qd0 : Inport  Port=2
  Add : Sum
  Add1 : Sum
  Demux : Demux  Outputs=3
  Demux1 : Demux  Outputs=3
  Gain : Gain  Gain=1/motor.lslb
  Gain1 : Gain  Gain=1/motor.lrlb
  Gain2 : Gain  Gain=motor.Mb
  Gain3 : Gain  Gain=motor.Mb
  Terminator : Terminator
  Terminator1 : Terminator
  Phi_m_q : Outport  VectorParamsAs1DForOutWhenUnconnected=off
  Phi_m_d : Outport  Port=2  VectorParamsAs1DForOutWhenUnconnected=off
  wires:
  Phi_s_qd0/1 -> Gain/1
  Demux/3 -> Terminator/1
  Demux1/3 -> Terminator1/1
  Phi_r_qd0/1 -> Gain1/1
  Gain/1 -> Demux/1
  Gain1/1 -> Demux1/1
  Add/1 -> Gain2/1
  Add1/1 -> Gain3/1
  Gain2/1 -> Phi_m_q/1
  Gain3/1 -> Phi_m_d/1
  Demux/1 -> Add/1
  Demux1/1 -> Add/2
  Demux/2 -> Add1/1
  Demux1/2 -> Add1/2

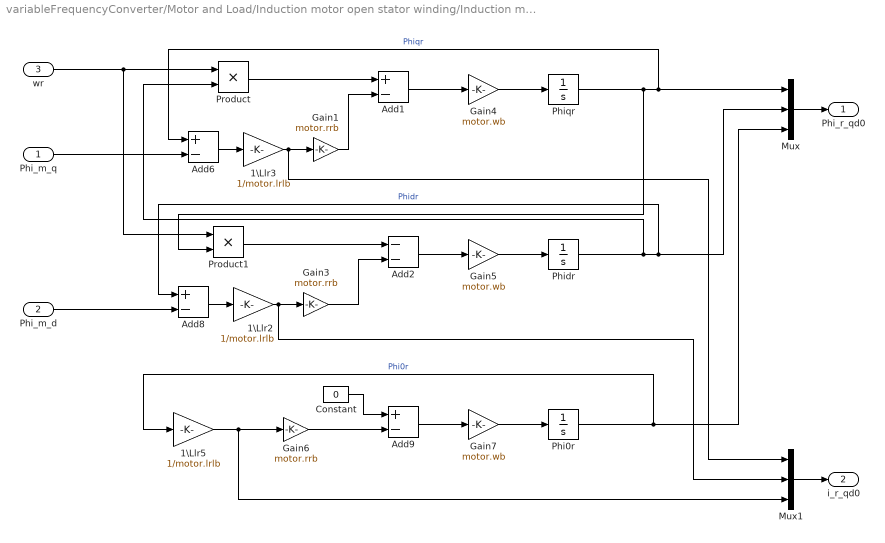
== system variableFrequencyConverter/Motor and Load/Induction motor open stator winding/Induction motor model/Rotor ==
  Phi_m_q : Inport
  Phi_m_d : Inport  Port=2
  wr : Inport  Port=3
  1\Llr2 : Gain  Gain=1/motor.lrlb  SaturateOnIntegerOverflow=on  OutDataTypeStr=Inherit: Same as input  ParamDataTypeStr=Inherit: Same as input
  1\Llr3 : Gain  Gain=1/motor.lrlb  SaturateOnIntegerOverflow=on  OutDataTypeStr=Inherit: Same as input  ParamDataTypeStr=Inherit: Same as input
  1\Llr5 : Gain  Gain=1/motor.lrlb  SaturateOnIntegerOverflow=on  OutDataTypeStr=Inherit: Same as input  ParamDataTypeStr=Inherit: Same as input
  Add{1,6,8..9} (4 alike) : Sum  Inputs=+-
  Add2 : Sum  Inputs=--
  Constant : Constant  Value=0
  Gain1 : Gain  Gain=motor.rrb
  Gain3 : Gain  Gain=motor.rrb
  Gain4 : Gain  Gain=motor.wb
  Gain5 : Gain  Gain=motor.wb
  Gain6 : Gain  Gain=motor.rrb
  Gain7 : Gain  Gain=motor.wb
  Mux : Mux  Inputs=3
  Mux1 : Mux  Inputs=3
  Phi0r : Integrator
  Phidr : Integrator
  Phiqr : Integrator
  Product : Product  RndMeth=Zero
  Product1 : Product  RndMeth=Zero
  Phi_r_qd0 : Outport  VectorParamsAs1DForOutWhenUnconnected=off
  i_r_qd0 : Outport  Port=2  VectorParamsAs1DForOutWhenUnconnected=off
  wires:
  wr/1 -> Product/1, Product1/1
  Phiqr/1 -> Product1/2, Add6/1, Mux/1  "Phiqr"
  Product/1 -> Add1/1
  Gain1/1 -> Add1/2
  Add1/1 -> Gain4/1
  Product1/1 -> Add2/1
  Gain3/1 -> Add2/2
  Add2/1 -> Gain5/1
  Phidr/1 -> Product/2, Add8/1, Mux/2  "Phidr"
  Phi0r/1 -> 1\Llr5/1, Mux/3  "Phi0r"
  Add8/1 -> 1\Llr2/1
  1\Llr2/1 -> Gain3/1, Mux1/2
  Add6/1 -> 1\Llr3/1
  1\Llr3/1 -> Gain1/1, Mux1/1
  1\Llr5/1 -> Gain6/1, Mux1/3
  Gain6/1 -> Add9/2
  Constant/1 -> Add9/1
  Add9/1 -> Gain7/1
  Phi_m_q/1 -> Add6/2
  Phi_m_d/1 -> Add8/2
  Mux/1 -> Phi_r_qd0/1
  Mux1/1 -> i_r_qd0/1
  Gain4/1 -> Phiqr/1
  Gain5/1 -> Phidr/1
  Gain7/1 -> Phi0r/1

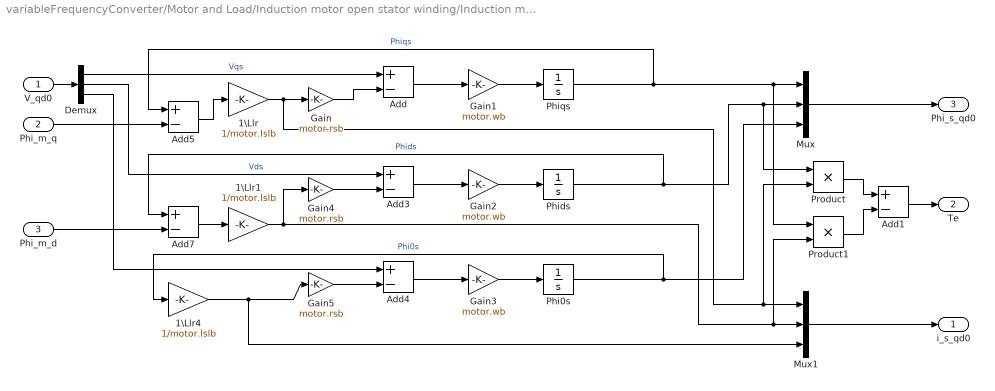
== system variableFrequencyConverter/Motor and Load/Induction motor open stator winding/Induction motor model/Stator ==
  V_qd0 : Inport
  Phi_m_q : Inport  Port=2
  Phi_m_d : Inport  Port=3
  1\Llr : Gain  Gain=1/motor.lslb  SaturateOnIntegerOverflow=on  OutDataTypeStr=Inherit: Same as input  ParamDataTypeStr=Inherit: Same as input
  1\Llr1 : Gain  Gain=1/motor.lslb  SaturateOnIntegerOverflow=on  OutDataTypeStr=Inherit: Same as input  ParamDataTypeStr=Inherit: Same as input
  1\Llr4 : Gain  Gain=1/motor.lslb  SaturateOnIntegerOverflow=on  OutDataTypeStr=Inherit: Same as input  ParamDataTypeStr=Inherit: Same as input
  Add{,1,3..5,7} (6 alike) : Sum  Inputs=+-
  Demux : Demux  Outputs=3
  Gain : Gain  Gain=motor.rsb
  Gain1 : Gain  Gain=motor.wb
  Gain2 : Gain  Gain=motor.wb
  Gain3 : Gain  Gain=motor.wb
  Gain4 : Gain  Gain=motor.rsb
  Gain5 : Gain  Gain=motor.rsb
  Mux : Mux  Inputs=3
  Mux1 : Mux  Inputs=3
  Phi0s : Integrator
  Phids : Integrator
  Phiqs : Integrator
  Product : Product  RndMeth=Zero
  Product1 : Product  RndMeth=Zero
  i_s_qd0 : Outport  VectorParamsAs1DForOutWhenUnconnected=off
  Te : Outport  Port=2  VectorParamsAs1DForOutWhenUnconnected=off
  Phi_s_qd0 : Outport  Port=3  VectorParamsAs1DForOutWhenUnconnected=off
  wires:
  V_qd0/1 -> Demux/1
  Demux/1 -> Add/1  "Vqs"
  Add/1 -> Gain1/1
  Gain/1 -> Add/2
  Phiqs/1 -> Add5/1, Mux/1, Product1/1  "Phiqs"
  Demux/2 -> Add3/1  "Vds"
  Gain4/1 -> Add3/2
  Add3/1 -> Gain2/1
  Phids/1 -> Add7/1, Mux/2, Product/1  "Phids"
  Demux/3 -> Add4/1
  1\Llr4/1 -> Gain5/1, Mux1/3
  Gain5/1 -> Add4/2
  Add4/1 -> Gain3/1
  Phi0s/1 -> 1\Llr4/1, Mux/3  "Phi0s"
  1\Llr/1 -> Mux1/1, Product/2, Gain/1
  Phi_m_q/1 -> Add5/2
  Add5/1 -> 1\Llr/1
  Phi_m_d/1 -> Add7/2
  Add7/1 -> 1\Llr1/1
  1\Llr1/1 -> Gain4/1, Mux1/2, Product1/2
  Mux/1 -> Phi_s_qd0/1
  Mux1/1 -> i_s_qd0/1
  Product1/1 -> Add1/2
  Product/1 -> Add1/1
  Add1/1 -> Te/1
  Gain1/1 -> Phiqs/1
  Gain2/1 -> Phids/1
  Gain3/1 -> Phi0s/1

== system variableFrequencyConverter/Motor and Load/Induction motor open stator winding/Induction motor model/abc => qdo stationary reference frame ==
  abc : Inport
  Constant : Constant  Value=0
  Demux : Demux  Outputs=3
  Gain : Gain  Gain=1/(sqrt(2)*motor.un)
  Mux : Mux  Inputs=3
  Mux2 : Mux  Inputs=2
  Trigonometric Function : Trigonometry
  Trigonometric Function1 : Trigonometry  Operator=cos
  abc_to_dq0 Transformation : powerlib_extras/Measurements/abc_to_dq0 Transformation
      settings: SourceProductBaseCode=PS
  qdo : Outport  VectorParamsAs1DForOutWhenUnconnected=off
  wires:
  Mux2/1 -> abc_to_dq0 Transformation/2
  abc/1 -> abc_to_dq0 Transformation/1
  abc_to_dq0 Transformation/1 -> Demux/1
  Mux/1 -> Gain/1
  Trigonometric Function/1 -> Mux2/1
  Trigonometric Function1/1 -> Mux2/2
  Gain/1 -> qdo/1
  Constant/1 -> Trigonometric Function/1, Trigonometric Function1/1
  Demux/1 -> Mux/2
  Demux/2 -> Mux/1
  Demux/3 -> Mux/3

== system variableFrequencyConverter/Motor and Load/Induction motor open stator winding/Induction motor model/qdo => abc stationary reference frame ==
  qdo : Inport
  Constant : Constant  Value=0
  Demux1 : Demux  Outputs=3
  Gain : Gain  Gain=sqrt(2)*motor.in
  Mux : Mux  Inputs=3
  Mux2 : Mux  Inputs=2
  Trigonometric Function : Trigonometry
  Trigonometric Function1 : Trigonometry  Operator=cos
  dq0_to_abc Transformation : powerlib_extras/Measurements/dq0_to_abc Transformation
      settings: SourceProductBaseCode=PS
  abc : Outport  VectorParamsAs1DForOutWhenUnconnected=off
  wires:
  Mux2/1 -> dq0_to_abc Transformation/2
  dq0_to_abc Transformation/1 -> abc/1
  qdo/1 -> Demux1/1
  Mux/1 -> Gain/1
  Constant/1 -> Trigonometric Function/1, Trigonometric Function1/1
  Trigonometric Function/1 -> Mux2/1
  Trigonometric Function1/1 -> Mux2/2
  Gain/1 -> dq0_to_abc Transformation/1
  Demux1/1 -> Mux/2
  Demux1/2 -> Mux/1
  Demux1/3 -> Mux/3

== system variableFrequencyConverter/Variable Frequency Converter/Controller/ControlProcess/Sine // Saddle PWM ==
  freqDes : Inport
  Enable : EnablePort
  Mux : Mux  Inputs=3
  Sine Saddle pulse width modulation : MATLAB Function  TreatAsAtomicUnit=on
  ccrValues : Outport  InitialOutput=ctrl.timerARR/2  VectorParamsAs1DForOutWhenUnconnected=off
  wires:
  freqDes/1 -> Sine Saddle pulse width modulation/1(freqDes)
  Mux/1 -> ccrValues/1
  Sine Saddle pulse width modulation/1(ccrA) -> Mux/1
  Sine Saddle pulse width modulation/2(ccrB) -> Mux/2
  Sine Saddle pulse width modulation/3(ccrC) -> Mux/3

== system variableFrequencyConverter/Variable Frequency Converter/Controller/ControlProcess/Space Vector PWM ==
  freqDes : Inport
  Enable : EnablePort
  Mux : Mux  Inputs=3
  Space vector pulse width modulation : MATLAB Function  TreatAsAtomicUnit=on
  ccrValues : Outport  InitialOutput=ctrl.timerARR/2  VectorParamsAs1DForOutWhenUnconnected=off
  wires:
  freqDes/1 -> Space vector pulse width modulation/1(freqDes)
  Space vector pulse width modulation/3(ccrC) -> Mux/3
  Space vector pulse width modulation/2(ccrB) -> Mux/2
  Mux/1 -> ccrValues/1
  Space vector pulse width modulation/1(ccrA) -> Mux/1

== system variableFrequencyConverter/Variable Frequency Converter/Controller/ControlProcess/Start ramp generator ==
  filtCurrent : Inport
  " " : simulink/Logic and Bit Operations/Compare To Constant  relop=>=  const=ctrl.currentLimitFactor*motor.In*sqrt(2)  OutDataTypeStr=boolean
  "  " : Logic  Operator=NOT  AllPortsSameDT=off  OutDataTypeStr=boolean
  Abs : Abs
  Add : Sum
  Constant1 : Constant  Value=ctrl.startRamp.inc
  Demux : Demux  Outputs=3
  MinMax : MinMax  Function=max  Inputs=3
  Product : Product  RndMeth=Zero
  Saturation : Saturate  UpperLimit=1  LowerLimit=0  ZeroCross=off
  Unit Delay : UnitDelay  SampleTime=-1  HasFrameUpgradeWarning=on
  ref : Outport  InitialOutput=0  VectorParamsAs1DForOutWhenUnconnected=off
  wires:
  Saturation/1 -> ref/1
  Unit Delay/1 -> Add/2
  Product/1 -> Add/1
  Add/1 -> Saturation/1, Unit Delay/1
  Constant1/1 -> Product/1
  Abs/1 -> Demux/1
  Demux/3 -> MinMax/3
  Demux/2 -> MinMax/2
  Demux/1 -> MinMax/1
  MinMax/1 -> " "/1
  "  "/1 -> Product/2
  " "/1 -> "  "/1
  filtCurrent/1 -> Abs/1

== system variableFrequencyConverter/Variable Frequency Converter/Controller/ControlProcess/Stop ramp generator ==
  Enable : EnablePort
  Add : Sum
  Add1 : Sum  Inputs=+-
  Constant1 : Constant  Value=ctrl.stopRamp.dec
  Constant2 : Constant
  Saturation : Saturate  UpperLimit=1  LowerLimit=0  ZeroCross=off
  Unit Delay : UnitDelay  SampleTime=-1  HasFrameUpgradeWarning=on
  ref : Outport  InitialOutput=0  VectorParamsAs1DForOutWhenUnconnected=off
  wires:
  Saturation/1 -> ref/1
  Unit Delay/1 -> Add/2
  Constant1/1 -> Add/1
  Add/1 -> Unit Delay/1, Add1/2
  Constant2/1 -> Add1/1
  Add1/1 -> Saturation/1

== system variableFrequencyConverter/Variable Frequency Converter/Controller/ControlProcess/Top of ramp ==
  time : Inport
  Enable : EnablePort  PropagateVarSize=During execution  ShowOutputPort=on
  Add : Sum  Inputs=+-
  Constant2 : Constant
  Detect Rise Positive : simulink/Logic and Bit Operations/Detect Rise Positive  vinit=0  OutDataTypeStr=uint8
  Relational Operator : RelationalOperator  OutDataTypeStr=boolean  RndMeth=Nearest
  Sample & Hold3 : powerlib_extras/Control  Blocks/Sample & Hold  ic=0
      settings: SourceProductBaseCode=PS
  finished : Outport  OutputWhenDisabled=reset  InitialOutput=[0]  VectorParamsAs1DForOutWhenUnconnected=off
  wires:
  Sample & Hold3/1 -> Add/2
  Constant2/1 -> Relational Operator/2
  Detect Rise Positive/1 -> Sample & Hold3/2
  time/1 -> Sample & Hold3/1, Add/1
  Enable/1 -> Detect Rise Positive/1
  Add/1 -> Relational Operator/1
  Relational Operator/1 -> finished/1

== matlab function variableFrequencyConverter/Variable Frequency Converter/Controller/PwmDriver/gateSignalGenerator ==
  data: T1 output; T2 output; T3 output; T4 output; T5 output; T6 output; pwmIn1 input; pwmIn2 input; pwmIn3 input
function [T1,T2,T3,T4,T5,T6] = gateSignalGenerator(pwmIn1, pwmIn2, pwmIn3)

if (pwmIn1) 
    T1 = 1;
    T2 = 0;
else
    T1 = 0;
    T2 = 1;
end

if (pwmIn2) 
    T3 = 1;
    T4 = 0;
else
    T3 = 0;
    T4 = 1;
end

if (pwmIn3) 
    T5 = 1;
    T6 = 0;
else
    T5 = 0;
    T6 = 1;
end

% Prevent SC
if (T1 && T2)
   T1 = 0;
   T2 = 0;
end

if (T3 && T4)
   T3 = 0;
   T4 = 0;
end

if (T5 && T6)
   T5 = 0;
   T6 = 0;
end

== matlab function variableFrequencyConverter/Variable Frequency Converter/Controller/ControlProcess/Selection ==
  data: spaceVectorPWM output; method input; sineSaddlePWM output
function [spaceVectorPWM,sineSaddlePWM] = selection(method)

if (method == 1 || method == 2)
    sineSaddlePWM = 1;
    spaceVectorPWM = 0;
elseif (method == 3)
    sineSaddlePWM = 0;
    spaceVectorPWM = 1;
else
    sineSaddlePWM = 0;
    spaceVectorPWM = 0;
end

end

== matlab function variableFrequencyConverter/Variable Frequency Converter/Controller/ControlProcess/Sine // Saddle PWM/Sine Saddle pulse width modulation ==
  data: freqDes input; ccrA output; ccrB output; ccrC output; ctrl parameter
function [ccrA,ccrB,ccrC] = sineSaddlePulseWidthModulation(freqDes, ctrl)
% Generate Sine or Saddle waveforms using a linear Volts per Hertz profile

persistent t_cnt

if isempty (t_cnt)
    t_cnt = 0;
end

TWO_PI = 2*pi;
TWO_DIV_SQRT_THREE = 2/sqrt(3);

if (ctrl.method == 1)  % Sine
    slope = 1 / ctrl.freqNom;
else  % Saddle
    slope = TWO_DIV_SQRT_THREE / ctrl.freqNom;
end

% Open loop Volts per Hertz control
f_des = freqDes * ctrl.freqNom;
v_des = slope * f_des;

if (f_des < ctrl.minFrequency)
    f_des = ctrl.minFrequency;
end

% Calculate number of executions corresponding to the desired frequency
period_cnt = round(1/(f_des*ctrl.deltaControlProcess));

% reference angle for the three phase sine waves
phi = TWO_PI * ctrl.deltaControlProcess * f_des * t_cnt;

% wrap the counter at every end of the period
t_cnt = t_cnt + 1;
if (t_cnt >= period_cnt)
    t_cnt = 0;
end

% phase a angle
phase_a_angle = phi;
if (phase_a_angle > TWO_PI) 
    phase_a_angle = phase_a_angle - TWO_PI;
elseif (phase_a_angle < 0) 
    phase_a_angle = phase_a_angle + TWO_PI;
else
    % no change in the value of phase_a_angle
end

% phase b angle is shifted 2*PI/3 radians (120 degrees)
phase_b_angle = phi - (TWO_PI/3);
if (phase_b_angle > TWO_PI) 
    phase_b_angle = phase_b_angle - TWO_PI;
elseif (phase_b_angle < 0) 
    phase_b_angle = phase_b_angle + TWO_PI;
else
    % no change in the value of phase_b_angle
end

% phase b angle is shifted 4*PI/3 radians (240 degrees)
phase_c_angle = phi - ((2*TWO_PI)/3);
if (phase_c_angle > TWO_PI) 
    phase_c_angle = phase_c_angle - TWO_PI;
elseif (phase_c_angle < 0) 
    phase_c_angle = phase_c_angle + TWO_PI;
else
    % no change in the value of phase_c_angle
end

if (ctrl.method == 1)  % Sine
    va = v_des * sin(phase_a_angle);
    vb = v_des * sin(phase_b_angle);
    vc = v_des * sin(phase_c_angle);
else  % Saddle
    v_des_third_harmonic = v_des / 6;
    va3 = v_des_third_harmonic*sin(3*phase_a_angle);
    vb3 = v_des_third_harmonic*sin(3*phase_b_angle);
    vc3 = v_des_third_harmonic*sin(3*phase_c_angle);
    va = v_des * sin(phase_a_angle) + va3;
    vb = v_des * sin(phase_b_angle) + vb3;
    vc = v_des * sin(phase_c_angle) + vc3;
end

% Convert to us
ccrA = ((va + 1) / 2) * ctrl.timerARR;
if (ctrl.rotationDirection == 1)  % Forward
    ccrB = ((vb + 1) / 2) * ctrl.timerARR;
    ccrC = ((vc + 1) / 2) * ctrl.timerARR;
else  % Reverse
    ccrB = ((vc + 1) / 2) * ctrl.timerARR;
    ccrC = ((vb + 1) / 2) * ctrl.timerARR;
end

== matlab function variableFrequencyConverter/Variable Frequency Converter/Controller/ControlProcess/Space Vector PWM/Space vector pulse width modulation ==
  data: freqDes input; ccrA output; ccrB output; ccrC output; ctrl parameter
function [ccrA, ccrB, ccrC] = spaceVectorPulseWidthModulation(freqDes, ctrl)
% Generate space vector waveforms using a linear Volts per Hertz profile

PHI_DIV_THREE = pi / 3;

persistent k
persistent phi_p

if isempty (k)
    k = 1;
    phi_p = 0;
end

% Open loop Voltz per Hertz control
slope = 1 / ctrl.freqNom;
f_des = freqDes * ctrl.freqNom;
v_des = slope * f_des;
if (f_des < ctrl.minFrequency)
   f_des = ctrl.minFrequency;
end

phi_p = (2 * pi * f_des * ctrl.deltaControlProcess) + phi_p;

if (phi_p >= PHI_DIV_THREE)
    phi_p = phi_p - PHI_DIV_THREE;
    
    % Determine sector
    k = k + 1;
    if (k > 6)
        k = 1;
    end
end

phi_p_p = PHI_DIV_THREE - phi_p;

d_a = v_des * sin(phi_p);
d_b = v_des * sin(phi_p_p);

switch (k)
    case 1
        c_a = -d_a - d_b;
        c_b = -d_a + d_b;
        c_c = d_a + d_b;
    case 2
        c_a = d_a - d_b;
        c_b = -d_a - d_b;
        c_c = d_a + d_b;        
    case 3
        c_a = d_a + d_b;
        c_b = -d_a - d_b;
        c_c = -d_a + d_b;         
    case 4
        c_a = d_a + d_b;
        c_b = d_a - d_b;
        c_c = -d_a - d_b;           
    case 5
        c_a = -d_a + d_b;
        c_b = d_a + d_b;
        c_c = -d_a - d_b;         
    case 6
        c_a = -d_a - d_b;
        c_b = d_a + d_b;
        c_c = d_a - d_b;       
    otherwise
        c_a = 0;
        c_b = 0;
        c_c = 0;
end

% Calculate compare register values
ccr_a = (1 + c_a) / (4 * ctrl.pwmFrequency);
ccr_b = (1 + c_b) / (4 * ctrl.pwmFrequency);
ccr_c = (1 + c_c) / (4 * ctrl.pwmFrequency);

% Convert to us
ccrA = ccr_a * 1e6;
if (ctrl.rotationDirection == 1)  % Forward
    ccrB = ccr_b * 1e6;
    ccrC = ccr_c * 1e6;
else  % Reverse
    ccrB = ccr_c * 1e6;
    ccrC = ccr_b * 1e6;
end

== matlab function variableFrequencyConverter/Variable Frequency Converter/Controller/ControlProcess/IIR Filter ==
  data: x1 input; x2 input; x3 input; y1 output; ctrl parameter; y2 output; y3 output
function [y1, y2, y3] = iirFilter(x1, x2, x3, ctrl)
% Infinite impulse response filter

FILTER_FREQUENCY = 100;  %[Hz]

% Filter coefficient
FILT_K = ctrl.deltaControlProcess / ((1/(2*pi*FILTER_FREQUENCY)) + ctrl.deltaControlProcess);

% The persistent variables are retained in memory before calls to the function
persistent y1Prev;
persistent y2Prev;
persistent y3Prev;

% Initialize the persistent variables
if isempty(y1Prev)
    y1Prev = 0;
    y2Prev = 0;
    y3Prev = 0;
end

y1 = (1 - FILT_K) * y1Prev + FILT_K * x1;
y1Prev = y1;

y2 = (1 - FILT_K) * y2Prev + FILT_K * x2;
y2Prev = y2;

y3 = (1 - FILT_K) * y3Prev + FILT_K * x3;
y3Prev = y3;

end
